simulink model "joystick_prueba"  (R2021a)
settings: Solver=VariableStepAuto  StartTime=0.0  StopTime=inf  RelTol=1e-3
libraries: vrlib x1
settings Model: Creator=agustin  LastModifiedBy=agustin

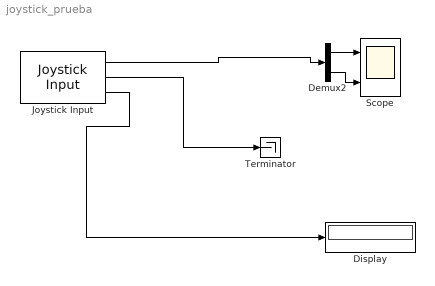
== system joystick_prueba ==
  Demux2 : Demux  Outputs=2
  Display : Display
  Joystick Input : vrlib/Joystick Input  joyid=1  adjustports=on  forcefeed=off
  Scope : Scope  NumInputPorts=2
  Terminator : Terminator
  wires:
  Joystick Input/1 -> Demux2/1
  Joystick Input/2 -> Terminator/1
  Joystick Input/3 -> Display/1
  Demux2/2 -> Scope/2
  Demux2/1 -> Scope/1
